simulink model "CalculateFloatingSystem"  (R2016b)
settings: Solver=VariableStepAuto  StartTime=0.0  StopTime=10.0  RelTol=1e-3
settings Model: Creator=NEATdemo  LastModifiedBy=NEATdemo

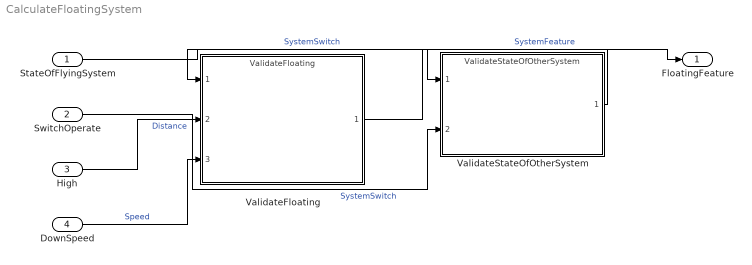
== system CalculateFloatingSystem ==
  StateOfFlyingSystem : Inport
      settings: AttributesFormatString=SystemSwitch
  SwitchOperate : Inport  Port=2
      settings: AttributesFormatString=SystemSwitch
  High : Inport  Port=3
      settings: AttributesFormatString=Distance
  DownSpeed : Inport  Port=4
      settings: AttributesFormatString=Speed
  ValidateFloating : ModelReference  ModelNameDialog=ValidateFloating  SimulationMode=Normal  ModelReferenceVersion=1.5
  ValidateStateOfOtherSystem : ModelReference  ModelNameDialog=ValidateStateOfOtherSystem  SimulationMode=Normal  ModelReferenceVersion=1.4
  FloatingFeature : Outport
      settings: AttributesFormatString=SystemFeature
  wires:
  ValidateStateOfOtherSystem/1 -> ValidateFloating/1
  StateOfFlyingSystem/1 -> ValidateStateOfOtherSystem/1  "SystemSwitch"
  SwitchOperate/1 -> ValidateStateOfOtherSystem/2  "SystemSwitch"
  High/1 -> ValidateFloating/2  "Distance"
  DownSpeed/1 -> ValidateFloating/3  "Speed"
  ValidateFloating/1 -> FloatingFeature/1  "SystemFeature"
